simulink model "stb_disc_sat"  (Simulink 5.0)
settings: Solver=ode15s  StartTime=t_init  StopTime=t_final  RelTol=1e-3
values from neighbouring files (symbols this model uses):
  B = zeros(1,degB+1)    [ext.m]
  C = [C Ck]    [polmul.m]
  D = D/D(1)    [tfvar.m]
undefined symbols (not defined in the file or in its folder): A, E, F, gamma, L, PSc, PTc, st, st1, st2, t_init2, Ts, U, zk
settings Model: Creator=kannan  LastModifiedBy=kannan  ExtModeAutoUpdateStatusClock=off

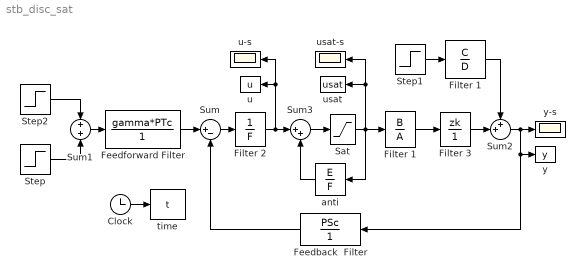
== system stb_disc_sat ==
  " Filter 1" : DiscreteFilter  Numerator=B  Denominator=A  SampleTime=Ts
  " Filter 2" : DiscreteFilter  Numerator=1  Denominator=F  SampleTime=Ts
  " Filter 3" : DiscreteFilter  Numerator=zk  Denominator=1  SampleTime=Ts
  " anti" : DiscreteFilter  Orientation=left  Numerator=E  Denominator=F  SampleTime=Ts
  Clock : Clock
      settings: Decimation=10
  Feedback  Filter : DiscreteFilter  Orientation=left  Numerator=PSc  Denominator=1  SampleTime=Ts
  Feedforward Filter : DiscreteFilter  Numerator=gamma*PTc  Denominator=1  SampleTime=Ts
  Filter 1 : DiscreteFilter  Numerator=C  Denominator=D  SampleTime=Ts
  Sat : Saturate  UpperLimit=U  LowerLimit=L
  Step : Step  Time=0  After=st  SampleTime=Ts
  Step1 : Step  Time=0  After=st1  SampleTime=Ts
  Step2 : Step  Time=t_init2  After=st2  SampleTime=Ts
  Sum : Sum  Inputs=|+-  SaturateOnIntegerOverflow=on
  Sum1 : Sum  Inputs=+|+  SaturateOnIntegerOverflow=on
  Sum2 : Sum  Inputs=++|  SaturateOnIntegerOverflow=on
  Sum3 : Sum  Inputs=|++  SaturateOnIntegerOverflow=on
  time : ToWorkspace  VariableName=t  SampleTime=Ts  SaveFormat=Array
  u : ToWorkspace  VariableName=u  SampleTime=Ts  SaveFormat=Array
  u-s : Scope
      settings: YMin=-20  YMax=20
  usat : ToWorkspace  VariableName=usat  SampleTime=Ts  SaveFormat=Array
  usat-s : Scope
      settings: YMin=-1.5  YMax=1.5  SaveName=ScopeData2
  y : ToWorkspace  VariableName=y  SampleTime=Ts  SaveFormat=Array
  y-s : Scope
      settings: YMin=-1.5  YMax=1.5
  wires:
  Feedforward Filter/1 -> Sum/1
  Feedback  Filter/1 -> Sum/2
  Clock/1 -> time/1
  Filter 1/1 -> Sum2/1
  Step1/1 -> Filter 1/1
  Sum2/1 -> y-s/1, Feedback  Filter/1, y/1
  Sum/1 -> " Filter 2"/1
  Sum1/1 -> Feedforward Filter/1
  " Filter 1"/1 -> " Filter 3"/1
  " Filter 3"/1 -> Sum2/2
  Sat/1 -> " Filter 1"/1, " anti"/1, usat-s/1, usat/1
  Step/1 -> Sum1/2
  Step2/1 -> Sum1/1
  " Filter 2"/1 -> Sum3/1, u-s/1, u/1
  Sum3/1 -> Sat/1
  " anti"/1 -> Sum3/2
